simulink library "subsea_glider_lib"  (R2024a)
settings: Solver=VariableStepAuto  StartTime=0.0  StopTime=10.0  RelTol=1e-3
undefined symbols (not defined in the file): AR, S
libraries: simulink x1
settings Model: Creator=Carson  LastModifiedBy=Carson

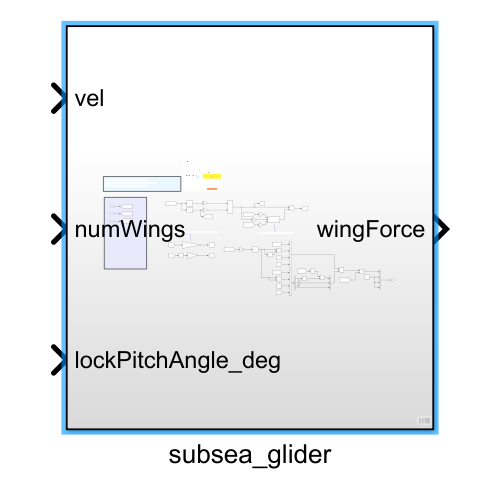
[thumbnail: Simulink's stored preview of the top-level diagram]
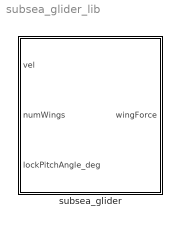
== system subsea_glider_lib ==
  subsea_glider : Subsystem

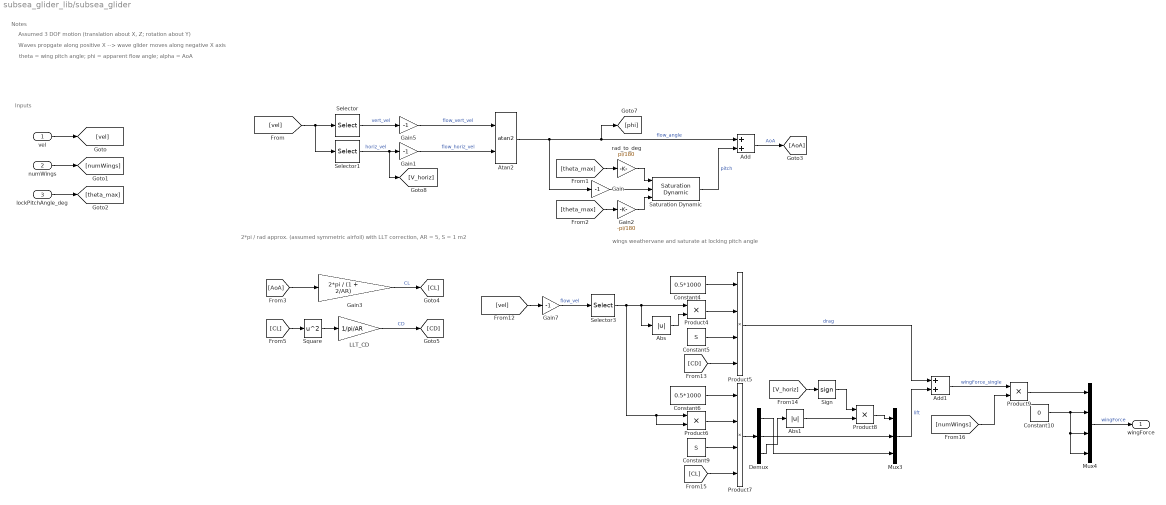
== system subsea_glider_lib/subsea_glider ==
  note: theta = wing pitch angle; phi = apparent flow angle; alpha = AoA
  note: Assumed 3 DOF motion (translation about X, Z; rotation about Y)
  note: Notes
  note: Inputs
  note: Waves propgate along positive X --> wave glider moves along negative X axis
  note: wings weathervane and saturate at locking pitch angle
  note: 2*pi / rad approx. (assumed symmetric airfoil) with LLT correction, AR = 5, S = 1 m2
  vel : Inport
  numWings : Inport  Port=2
  lockPitchAngle_deg : Inport  Port=3
  Abs : Abs  SaturateOnIntegerOverflow=off
  Abs1 : Abs  SaturateOnIntegerOverflow=off
  Add : Sum
  Add1 : Sum
  Atan2 : Trigonometry  Operator=atan2
  Constant10 : Constant  Value=0
  Constant4 : Constant  Value=0.5*1000
  Constant5 : Constant  Value=S
  Constant6 : Constant  Value=0.5*1000
  Constant9 : Constant  Value=S
  Demux : Demux  Outputs=3
  Gain{,1,5,7} (4 alike) : Gain  Gain=-1
  Gain2 : Gain  Gain=-pi/180
  Gain3 : Gain  Gain=2*pi / (1 + 2/AR)
  LLT_CD : Gain  Gain=1/pi/AR
  Mux3 : Mux  Inputs=3
  Mux4 : Mux
  Product{4,6,8..9} (4 alike) : Product
  Product5 : Product  Inputs=****
  Product7 : Product  Inputs=****
  Saturation Dynamic : simulink/Discontinuities/Saturation Dynamic  OutMin=[]  OutMax=[]  OutDataTypeStr=Inherit: Same as second input  OutDataType=fixdt(1, 16)  OutScaling=2^-10  DoSatur=off
  Selector : Selector  InputPortWidth=6  IndexOptions=Index vector (dialog)  Indices=3  OutputSizes=1
  Selector1 : Selector  InputPortWidth=6  IndexOptions=Index vector (dialog)  Indices=1  OutputSizes=1
  Selector3 : Selector  InputPortWidth=6  IndexOptions=Index vector (dialog)  Indices=[1 2 3]  OutputSizes=1
  Sign : Signum
  Square : Math  Operator=square
  rad_to_deg : Gain  Gain=pi/180
  wingForce : Outport
  wires:
  Mux4/1 -> wingForce/1  "wingForce"
  Constant10/1 -> Mux4/2, Mux4/3, Mux4/4
  Product9/1 -> Mux4/1
  [numWings] -> Product9/2
  Add1/1 -> Product9/1  "wingForce_single"
  Mux3/1 -> Add1/2  "lift"
  Product8/1 -> Mux3/1
  Sign/1 -> Product8/1
  [V_horiz] -> Sign/1
  Abs1/1 -> Product8/2
  Demux/3 -> Abs1/1
  Demux/1 -> Mux3/3
  Demux/2 -> Mux3/2
  vel/1 -> [vel]
  numWings/1 -> [numWings]
  lockPitchAngle_deg/1 -> [theta_max]
  [vel] -> Selector1/1, Selector/1
  Selector/1 -> Gain5/1  "vert_vel"
  Selector1/1 -> Gain1/1, [V_horiz]  "horiz_vel"
  Gain5/1 -> Atan2/1  "flow_vert_vel"
  Gain1/1 -> Atan2/2  "flow_horiz_vel"
  Atan2/1 -> Gain/1, [phi], Add/1  "flow_angle"
  Gain/1 -> Saturation Dynamic/2
  [theta_max] -> rad_to_deg/1
  [theta_max] -> Gain2/1
  Gain2/1 -> Saturation Dynamic/3
  Saturation Dynamic/1 -> Add/2  "pitch"
  Add/1 -> [AoA]  "AoA"
  rad_to_deg/1 -> Saturation Dynamic/1
  [AoA] -> Gain3/1
  Gain3/1 -> [CL]  "CL"
  [CL] -> Square/1
  Square/1 -> LLT_CD/1
  LLT_CD/1 -> [CD]  "CD"
  [vel] -> Gain7/1
  Abs/1 -> Product4/2
  Product4/1 -> Product5/2
  Constant4/1 -> Product5/1
  Constant5/1 -> Product5/3
  [CD] -> Product5/4
  Product5/1 -> Add1/1  "drag"
  Product7/1 -> Demux/1
  [CL] -> Product7/4
  Constant9/1 -> Product7/3
  Constant6/1 -> Product7/1
  Product6/1 -> Product7/2
  Selector3/1 -> Product6/2, Product6/1, Product4/1, Abs/1
  Gain7/1 -> Selector3/1  "flow_vel"
